simulink model "lab3"  (R2022a)
settings: Solver=VariableStepAuto  StartTime=0.0  StopTime=1000  RelTol=1e-3
undefined symbols (not defined in the file or in its folder): m, n
settings Model: Creator=Веточка  LastModifiedBy=Веточка

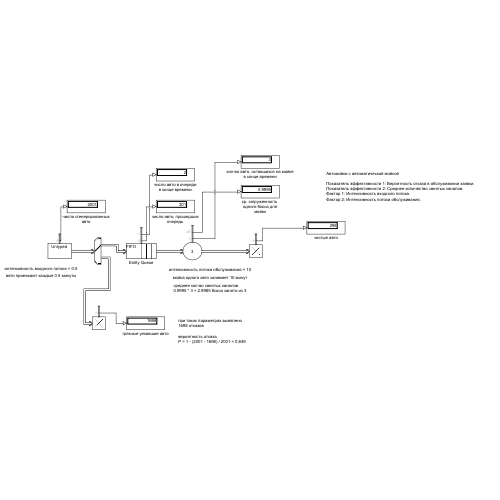
[thumbnail: Simulink's stored preview of the top-level diagram]
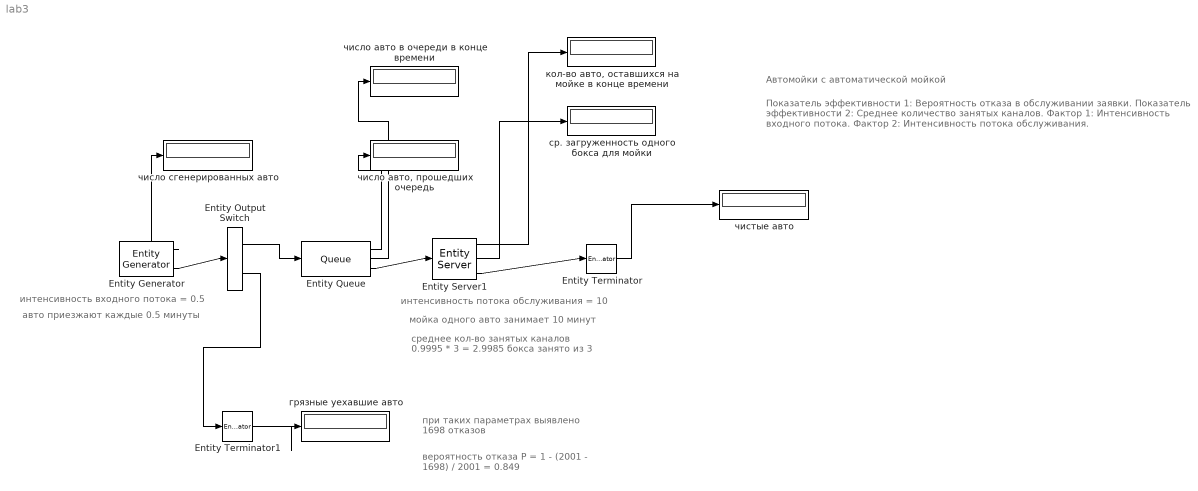
== system lab3 ==
  note: среднее кол-во занятых каналов
      | 0.9995 * 3 = 2.9985 бокса занято из 3
  note: вероятность отказа
      | Р = 1 - (2001 - 1698) / 2001 = 0.849
  note: при таких параметрах выявлено
      | 1698 отказов
  note: мойка одного авто занимает 10 минут
  note: интенсивность потока обслуживания = 10
  note: авто приезжают каждые 0.5 минуты
  note: интенсивность входного потока = 0.5
  note: Показатель эффективности 1: Вероятность отказа в обслуживании заявки. Показатель эффективности 2: Среднее количество занятых каналов.
      | Фактор 1: Интенсивность входного потока.
      | Фактор 2: Интенсивность потока обслуживания.
  note: Автомойки с автоматической мойкой
  Entity Output Switch : EntityOutputSwitch  InputPortMessageModes=m  OutputPortMessageModes=m,m  SwitchAttributeName=Attribute1
  Entity Generator : EntityGenerator  OutputPortMessageModes=n,m  Period=0.5  AttributeName=entity  AttributeInitialValue=0  NumberEntitiesDeparted=on  EntityTypeName=Entity
      settings: OutputPortMap=o0,o3
  Entity Queue : Queue  InputPortMessageModes=m  OutputPortMessageModes=n,n,m  Capacity=3  NumberEntitiesDeparted=on  NumberEntitiesInBlock=on
      settings: OutputPortMap=o0,o1,o5
  Entity Server1 : EntityServer  InputPortMessageModes=m  OutputPortMessageModes=n,n,m  Capacity=3  ServiceTimeValue=10  NumberEntitiesInBlock=on  Utilization=on
      settings: OutputPortMap=o1,o5,o9
  Entity Terminator : EntityTerminator  InputPortMessageModes=m  NumberEntitiesArrived=on
      settings: OutputPortMap=o0
  Entity Terminator1 : EntityTerminator  InputPortMessageModes=m  NumberEntitiesArrived=on
      settings: OutputPortMap=o0
  грязные уехавшие авто : Display
  "кол-во авто, оставшихся на мойке в конце времени" : Display
  ср. загруженность одного бокса для мойки : Display
  число авто в очереди в конце времени : Display
  "число авто, прошедших очередь" : Display
  число сгенерированных авто : Display
  чистые авто : Display
  wires:
  Entity Generator/1 -> число сгенерированных авто/1
  Entity Queue/1 -> "число авто, прошедших очередь"/1
  Entity Terminator/1 -> чистые авто/1
  Entity Server1/2 -> ср. загруженность одного бокса для мойки/1
  Entity Generator/2 -> Entity Output Switch/1
  Entity Output Switch/1 -> Entity Queue/1
  Entity Terminator1/1 -> грязные уехавшие авто/1
  Entity Output Switch/2 -> Entity Terminator1/1
  Entity Queue/3 -> Entity Server1/1
  Entity Server1/3 -> Entity Terminator/1
  Entity Server1/1 -> "кол-во авто, оставшихся на мойке в конце времени"/1
  Entity Queue/2 -> число авто в очереди в конце времени/1
